simulink model "lab3"  (R2017a)
settings: Solver=FixedStepDiscrete  StartTime=0.0  StopTime=inf  RelTol=1e-3
libraries: simulink x1, dsparch4 x1
settings Model: Creator=SashaBoss  LastModifiedBy=SashaBoss
settings SolverCC: AutoInsertRateTranBlk=on
settings DataIOCC: LimitDataPoints=on  SaveOutput=off  SignalLogging=off  SaveTime=off
settings OptimizationCC: LifeSpan=inf
settings DebuggingCC: AlgebraicLoopMsg=error  SingleTaskRateTransMsg=error  AllowSymbolicDim=off  SFUnexpectedBacktrackingDiag=warning  SFNoUnconditionalDefaultTransitionDiag=warning  SFExecutionAtInitializationDiag=none
settings GRTTargetCC: TargetLangStandard=C89/C90 (ANSI)  GeneratePreprocessorConditionals=Disable all

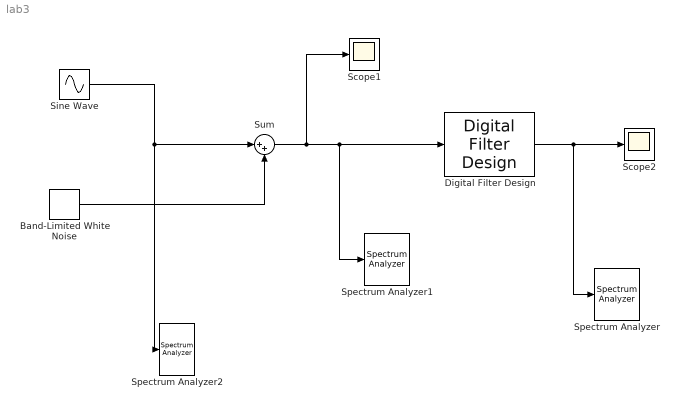
== system lab3 ==
  Band-Limited White Noise : simulink/Sources/Band-Limited White Noise  Cov=[0.08]  Ts=0.1  seed=[23341]
  Digital Filter Design : dsparch4/Digital Filter Design  mwdsp_browser_bugfix_var=off
  Scope1 : Scope
  Scope2 : Scope
  Sine Wave : Sin  SineType=Sample based  Samples=10000  SampleTime=0.01
  Spectrum Analyzer : SpectrumAnalyzer
  Spectrum Analyzer1 : SpectrumAnalyzer
  Spectrum Analyzer2 : SpectrumAnalyzer
  Sum : Sum  Inputs=|++
  wires:
  Sine Wave/1 -> Sum/1, Spectrum Analyzer2/1
  Band-Limited White Noise/1 -> Sum/2
  Sum/1 -> Scope1/1, Digital Filter Design/1, Spectrum Analyzer1/1
  Digital Filter Design/1 -> Spectrum Analyzer/1, Scope2/1
